simulink model "camera"  (R2017a)
settings: Solver=VariableStepAuto  StartTime=0.0  StopTime=inf  RelTol=1e-3
values from neighbouring files (symbols this model uses):
  C = [1 0 0]    [principal.m]
undefined symbols (not defined in the file or in its folder): IsPositionTracked, IsSkeletonTracked, JointDepthIndices, JointImageIndices, JointTrackingState, JointWorldCoordinates, none, PositionDepthIndices, PositionImageIndices, PositionWorldCoordinates, Rec, SDTV, SegmentationData, SkeletonTrackingID, strel, videoinput
libraries: simulink x6, visionsinks x3, visionstatistics x1, visionmorphops x1, visionconversions x1, visiontextngfix x1, imaqlib x1
settings Model: Creator=dscat  LastModifiedBy=dscat

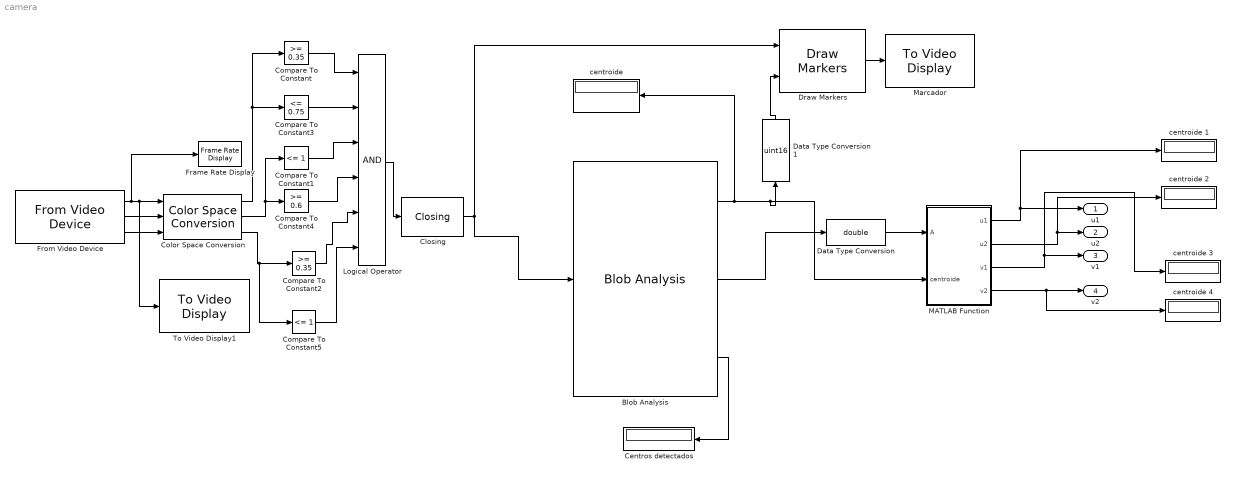
== system camera ==
  Blob Analysis : visionstatistics/Blob Analysis  Tag=vipblks_row_conv  area=off  centroid=on  bBox=off  majorAxis=off  minorAxis=off  angle=off  eccentricity=off  equivDiameterSq=off  extent=off  perimeter=on  maxBlobs=1  warnIfNumBlobsExceeded=on  isCount=on  useMinArea=on  minArea=20  useMaxArea=on  maxArea=60000000  excludeBorderBlob=off  outDT=double  isOutVarDim=off  isFill=on  fillValues=-1  conn=8  isLabel=off  outputMode=Binary point scaling  outputWordLength=32  outputFracLength=16  firstCoeffMode=Binary point scaling  firstCoeffWordLength=16  firstCoeffFracLength=14  secondCoeffMode=Binary point scaling  secondCoeffWordLength=32  secondCoeffFracLength=16  accumMode=Binary point scaling  accumWordLength=32  accumFracLength=0  prodOutputMode=Binary point scaling  prodOutputWordLength=32  prodOutputFracLength=16  roundingMode=Floor  overflowMode=off
      settings: SourceProductName=Computer Vision System Toolbox
  Centros detectados : Display
  Closing : visionmorphops/Closing  nhoodsrc=Specify via dialog  strel=strel('square',2)
      settings: SourceProductName=Computer Vision System Toolbox  SourceProductBaseCode=VP
  Color Space Conversion : visionconversions/Color Space  Conversion  conversion=Obsolete  conversionActive=R'G'B' to HSV  wp_str=D65  rec=Rec. 601 (SDTV)  sys=1125/60/2:1  imagePorts=Separate color signals
      settings: SourceProductName=Computer Vision System Toolbox
  Compare To Constant : simulink/Logic and Bit Operations/Compare To Constant  relop=>=  const=0.35  OutDataTypeStr=boolean
  Compare To Constant1 : simulink/Logic and Bit Operations/Compare To Constant  relop=<=  const=1  OutDataTypeStr=boolean
  Compare To Constant2 : simulink/Logic and Bit Operations/Compare To Constant  relop=>=  const=0.35  OutDataTypeStr=boolean
  Compare To Constant3 : simulink/Logic and Bit Operations/Compare To Constant  relop=<=  const=0.75  OutDataTypeStr=boolean
  Compare To Constant4 : simulink/Logic and Bit Operations/Compare To Constant  relop=>=  const=0.6  OutDataTypeStr=boolean
  Compare To Constant5 : simulink/Logic and Bit Operations/Compare To Constant  relop=<=  const=1  OutDataTypeStr=boolean
  Data Type Conversion : DataTypeConversion  OutMin=0  OutMax=640  OutDataTypeStr=double
  Data Type Conversion1 : DataTypeConversion  OutMin=0  OutMax=640  OutDataTypeStr=uint16
  Draw Markers : visiontextngfix/Draw Markers  shape=X-mark  size=3  fill=off  fillClrSource=Specify via dialog  display=Black  intensity=200  color=[200 100 100]  opacity=0.6  viewport=Entire image  antialiasing=off  inType=Obsolete  imagePorts=One multidimensional signal  prodOutputMode=Binary point scaling  prodOutputWordLength=32  prodOutputFracLength=14  memoryMode=Specify word length  memoryWordLength=16  memoryFracLength=15  roundingMode=Floor  overflowMode=off
      settings: SourceProductName=Computer Vision System Toolbox  SourceProductBaseCode=VP
  Frame Rate Display : visionsinks/Frame Rate Display  UpdateRate=10
      settings: SourceProductName=Computer Vision System Toolbox  SourceProductBaseCode=VP
  From Video Device : imaqlib/From Video Device  DeviceMenu=winvideo 1 (HP Wide Vision HD Camera)  Device=winvideo 2 (Trust Webcam)  ObjConstructor=videoinput('winvideo', 2)  VideoFormatMenu=YUY2_640x480  VideoFormat=YUY2_640x480  VideoSource=input1  ROIPosition=[0 0 480 640]  EnableHWTrigger=off  TriggerConfiguration=none/none  SampleTime=1/20  OutputPortsMode=Separate color signals  DataType=single  CanDoHWTrigger=no  ReturnedColorSpace=rgb  BlockHandle=6.0001  ROIWidth=640  ROIHeight=480  ROIColumn=0  ROIRow=0  EngXMLPath=C:\Program Files\MATLAB\R2017a\toolbox\imaq\imaq\private  DevXMLPath=C:\ProgramData\MATLAB\SupportPackages\R2017a\toolbox\imaq\supportpackages\genericvideo\adaptor\win64  EngLibPath=C:\Program Files\MATLAB\R2017a\toolbox\imaq\imaqblks\imaqmex\win64  ColorSpace=rgb  BayerSensorAlignment=grbg  AllMetadata=IsPositionTracked;IsSkeletonTracked;JointDepthIndices;JointImageIndices;JointTrackingState;JointWorldCoordinates;PositionDepthIndices;PositionImageIndices;PositionWorldCoordinates;SegmentationData;SkeletonTrackingID
      settings: SourceProductName=Image Acquisition Toolbox
  Logical Operator : Logic  Inputs=6  AllPortsSameDT=off  OutDataTypeStr=boolean
  MATLAB Function : MATLAB Function  TreatAsAtomicUnit=on
  Marcador : visionsinks/To Video Display  windowSizeMode=True size (1:1)  openAtMdlStart=on  fullScreen=off  videoWindowX=60  videoWindowY=50  saveWindowSize=off  videoWindowWidth=640  videoWindowHeight=480  inputColorFormat=RGB  inputType=Obsolete  imagePorts=One multidimensional signal  OutputDevice=On-screen video monitor  dataOrg=Column-major  isWindowOpen=on
      settings: SourceProductName=Computer Vision System Toolbox
  To Video Display1 : visionsinks/To Video Display  windowSizeMode=Normal  openAtMdlStart=on  fullScreen=off  videoWindowX=7  videoWindowY=116  saveWindowSize=off  videoWindowWidth=1019  videoWindowHeight=447  inputColorFormat=RGB  inputType=Obsolete  imagePorts=One multidimensional signal  OutputDevice=On-screen video monitor  dataOrg=Column-major  isWindowOpen=off
      settings: SourceProductName=Computer Vision System Toolbox
  centroide {,1..4} (5 alike) : Display
      centroide 1 settings: Decimation=4
      centroide 2 settings: Decimation=4
      centroide 3 settings: Decimation=4
      centroide 4 settings: Decimation=4
  u1 : Outport  SampleTime=0.05
  u2 : Outport  Port=2  SampleTime=0.05
  v1 : Outport  Port=3
  v2 : Outport  Port=4
  wires:
  Blob Analysis/2 -> Data Type Conversion/1
  Data Type Conversion1/1 -> Draw Markers/2
  Compare To Constant1/1 -> Logical Operator/3
  Data Type Conversion/1 -> MATLAB Function/1(A)
  Compare To Constant5/1 -> Logical Operator/6
  Color Space Conversion/1 -> Compare To Constant3/1, Compare To Constant/1
  Logical Operator/1 -> Closing/1
  From Video Device/2 -> Color Space Conversion/2
  Blob Analysis/1 -> "centroide "/1, MATLAB Function/2(centroide), Data Type Conversion1/1
  Compare To Constant/1 -> Logical Operator/1
  Compare To Constant2/1 -> Logical Operator/5
  Compare To Constant4/1 -> Logical Operator/4
  From Video Device/1 -> Frame Rate Display/1, To Video Display1/1, Color Space Conversion/1
  From Video Device/3 -> Color Space Conversion/3
  Draw Markers/1 -> Marcador/1
  MATLAB Function/1(u1) -> u1/1, centroide 1/1
  Color Space Conversion/2 -> Compare To Constant1/1, Compare To Constant4/1
  MATLAB Function/2(u2) -> u2/1, centroide 2/1
  MATLAB Function/4(v2) -> v2/1, centroide 4/1
  Closing/1 -> Blob Analysis/1, Draw Markers/1
  Color Space Conversion/3 -> Compare To Constant5/1, Compare To Constant2/1
  MATLAB Function/3(v1) -> v1/1, centroide 3/1
  Blob Analysis/3 -> Centros detectados/1
  Compare To Constant3/1 -> Logical Operator/2

== matlab function camera/MATLAB Function ==
  data: A input; u1 output; u2 output; v1 output; v2 output; centroide input
function [u1,u2,v1,v2] = fcn(A, centroide)

lado = A/4  ;
u1 = centroide(1)-(lado/2) - 320;
u2 = centroide(1)+(lado/2) - 320;
v1 = -centroide(2)-(lado/2) + 240;
v2 = -centroide(2)+(lado/2) + 240;
